simulink model "simu_no_lineal_con_observador_en_state_space"  (R2023b)
settings: Solver=VariableStepAuto  StartTime=0.0  StopTime=100  RelTol=1e-3
settings Model: Creator=PC  LastModifiedBy=q
settings DebuggingCC: UnconnectedInputMsg=warning  UnconnectedOutputMsg=warning  UnconnectedLineMsg=warning
settings ModelReferenceCC: EnableRefExpFcnMdlSchedulingChecks=on
settings RTWCC: DLArmComputeVersion=19.05

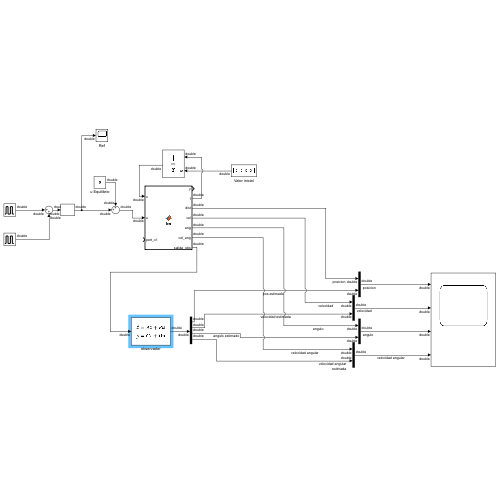
[thumbnail: Simulink's stored preview of the top-level diagram]
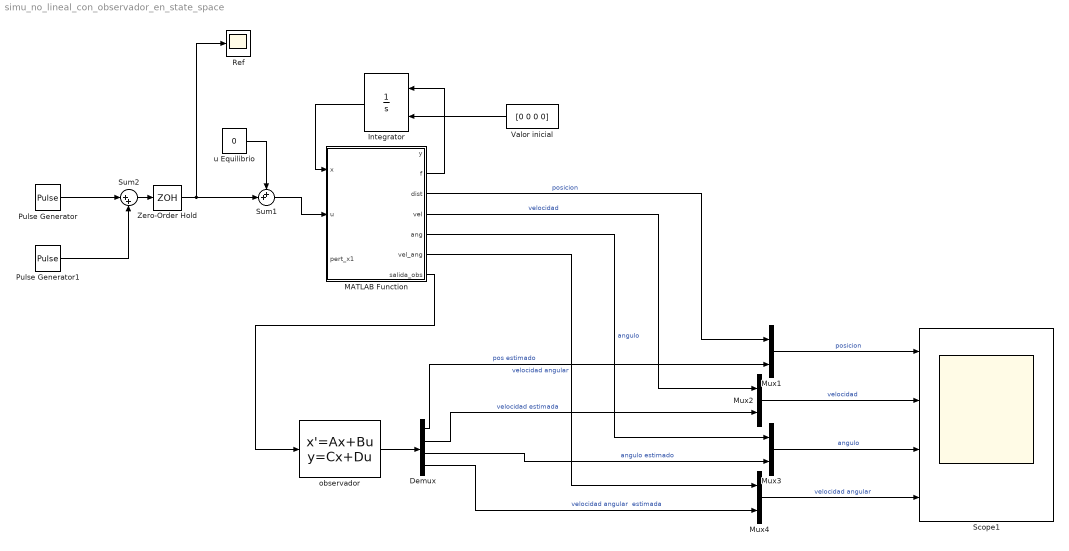
== system simu_no_lineal_con_observador_en_state_space ==
  Demux : Demux
  Integrator : Integrator  InitialConditionSource=external
  MATLAB Function : MATLAB Function  TreatAsAtomicUnit=on
  Mux{1..4} (4 alike) : Mux  Inputs=2
  Pulse Generator : DiscretePulseGenerator  PulseType=Time based  Amplitude=10*3.14/180  Period=10  PulseWidth=5  VectorParams1D=off
  Pulse Generator1 : DiscretePulseGenerator  PulseType=Time based  Amplitude=-10*3.14/180  Period=10  PulseWidth=5  PhaseDelay=5  VectorParams1D=off
  Ref : Scope
  Scope1 : Scope  NumInputPorts=4
  Sum1 : Sum  Inputs=++|
  Sum2 : Sum  Inputs=|++
  Valor inicial : Constant  Value=[0 0 0 0]
  Zero-Order Hold : ZeroOrderHold  SampleTime=0.02
  observador : StateSpace  A=[[1 0 0 0];[0 1 0 0];[0 0 1 0];[0 0 0 1]]  B=[1 0 1 0 ]'  C=[[1 0 0 0];[0 1 0 0];[0 0 1 0];[0 0 0 1]]  D=[0 0 0 0]'  InitialCondition=0
  u Equilibrio : Constant  Value=0
  wires:
  Valor inicial/1 -> Integrator/2
  MATLAB Function/2(f) -> Integrator/1
  u Equilibrio/1 -> Sum1/1
  Sum1/1 -> MATLAB Function/2(u)
  Integrator/1 -> MATLAB Function/1(x)
  observador/1 -> Demux/1
  MATLAB Function/6(vel_ang) -> Mux4/1  "velocidad angular"
  Demux/4 -> Mux4/2  "velocidad angular  estimada"
  Mux1/1 -> Scope1/1  "posicion"
  Demux/1 -> Mux1/2  "pos estimado"
  Mux2/1 -> Scope1/2  "velocidad"
  Mux4/1 -> Scope1/4  "velocidad angular"
  Demux/2 -> Mux2/2  "velocidad estimada"
  Demux/3 -> Mux3/2  "angulo estimado"
  MATLAB Function/5(ang) -> Mux3/1  "angulo"
  Mux3/1 -> Scope1/3  "angulo"
  MATLAB Function/4(vel) -> Mux2/1  "velocidad"
  MATLAB Function/3(dist) -> Mux1/1  "posicion"
  Pulse Generator/1 -> Sum2/1
  Pulse Generator1/1 -> Sum2/2
  Zero-Order Hold/1 -> Ref/1, Sum1/2
  Sum2/1 -> Zero-Order Hold/1
  MATLAB Function/7(salida_obs) -> observador/1

== matlab function simu_no_lineal_con_observador_en_state_space/MATLAB Function ==
  data: x input; u input; y output; f output; pert_x1 input; dist output; vel output; ang output; vel_ang output; salida_obs output
function [y, f,dist,vel,ang,vel_ang,salida_obs] = fcn(x, u, pert_x1)
    
    g = 9.81; %kg m/s2
    m = 0.047; %kg
    kv = 0.2;
    R = 0.02;
    mr = 0.00275;
    J = 0.5*4*mr*power(R,2);
    
    x(1) = x(1) + pert_x1;

    %Dinamica
    f1 = x(2);
    f2 = (m*g*sin(x(3)) - kv * x(2)) * 1/(m + (J/power(R,2)));
    f3 = x(4);
    f4 = -20.73 * x(4) - 154.47*x(3) + u * 64.89;

    y = x(1);
    f = [f1 f2 f3 f4];
    dist=x(1);
    vel=x(2);
    ang=x(3);
    vel_ang=x(4);
    salida_obs = [dist,ang];
end
